simulink model "tp1_simulink_h"  (R2024a)
settings: Solver=VariableStepAuto  StartTime=0.0  StopTime=10.0  RelTol=1e-3
values from neighbouring files (symbols this model uses):
  A = double(A)    [tp1_v2.m]
  B = double(B)    [tp1_v2.m]
  C = double(C)    [tp1_v2.m]
  D = double(D)    [tp1_v2.m]
  K = place(A, B, P)    [tp1_v2.m]
  kr = 1/k_dc    [tp1_v2.m]
  x0 = [1; 0; m*g]    [tp1_v2.m]
settings Model: Creator=tiago  LastModifiedBy=tiago

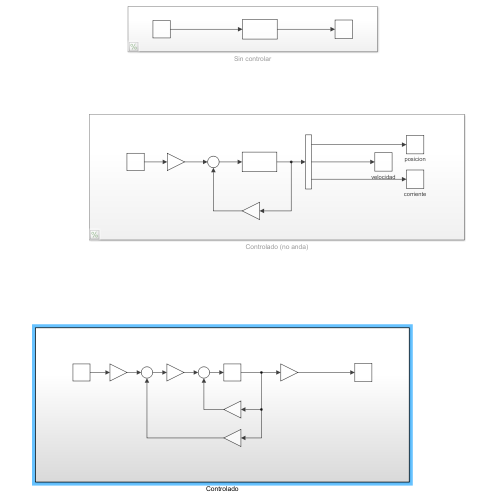
[thumbnail: Simulink's stored preview of the top-level diagram]
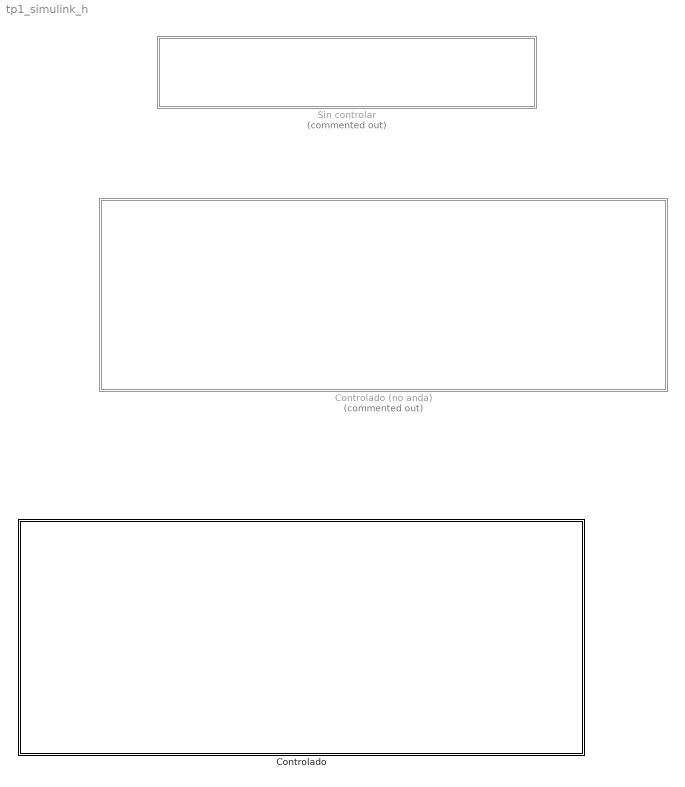
== system tp1_simulink_h ==
  Controlado : Subsystem
  Controlado (no anda) : Subsystem  Commented=on
  Sin controlar : Subsystem  Commented=on

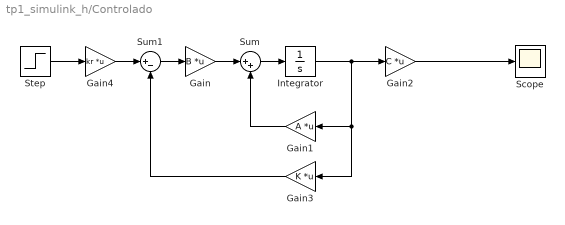
== system tp1_simulink_h/Controlado ==
  Gain : Gain  Gain=B  Multiplication=Matrix(K*u)
  Gain1 : Gain  Gain=A  Multiplication=Matrix(K*u)
  Gain2 : Gain  Gain=C  Multiplication=Matrix(K*u)
  Gain3 : Gain  Gain=K  Multiplication=Matrix(K*u)
  Gain4 : Gain  Gain=kr  Multiplication=Matrix(K*u)
  Integrator : Integrator
  Scope : Scope
  Step : Step  SampleTime=0
  Sum : Sum  Inputs=|++
  Sum1 : Sum  Inputs=|+-
  wires:
  Integrator/1 -> Gain3/1, Gain1/1, Gain2/1
  Gain2/1 -> Scope/1
  Gain3/1 -> Sum1/2
  Sum1/1 -> Gain/1
  Gain4/1 -> Sum1/1
  Step/1 -> Gain4/1
  Sum/1 -> Integrator/1
  Gain/1 -> Sum/1
  Gain1/1 -> Sum/2

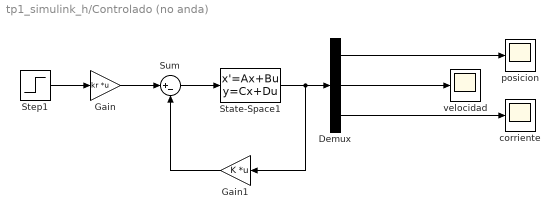
== system tp1_simulink_h/Controlado (no anda) ==
  Demux : Demux  Outputs=3
  Gain : Gain  Gain=kr  Multiplication=Matrix(K*u)
  Gain1 : Gain  Gain=K  Multiplication=Matrix(K*u)
  State-Space1 : StateSpace  A=A  B=B  C=[1 1 1]  D=D  InitialCondition=x0
  Step1 : Step  SampleTime=0
  Sum : Sum  Inputs=|+-
  corriente : Scope
  posicion : Scope
  velocidad : Scope
  wires:
  State-Space1/1 -> Gain1/1, Demux/1
  Gain1/1 -> Sum/2
  Demux/3 -> corriente/1
  Demux/2 -> velocidad/1
  Gain/1 -> Sum/1
  Sum/1 -> State-Space1/1
  Demux/1 -> posicion/1
  Step1/1 -> Gain/1

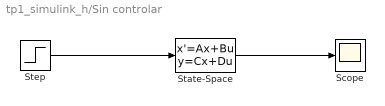
== system tp1_simulink_h/Sin controlar ==
  Scope : Scope
  State-Space : StateSpace  A=A  B=B  C=C  D=D  InitialCondition=x0
  Step : Step  SampleTime=0
  wires:
  Step/1 -> State-Space/1
  State-Space/1 -> Scope/1
